simulink model "model2"  (R2022b)
settings: Solver=VariableStepAuto  StartTime=0.0  StopTime=20  RelTol=1e-3
settings Model: Creator=jim  LastModifiedBy=jim

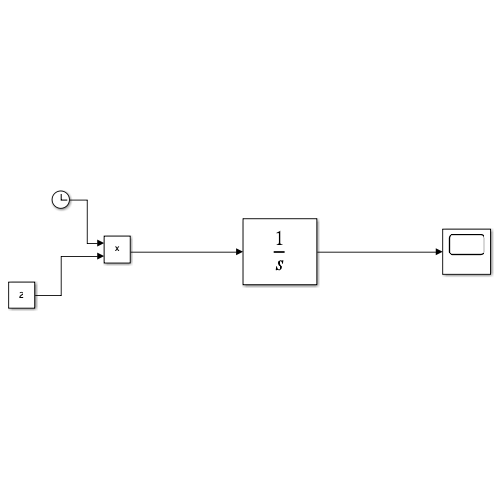
[thumbnail: Simulink's stored preview of the top-level diagram]
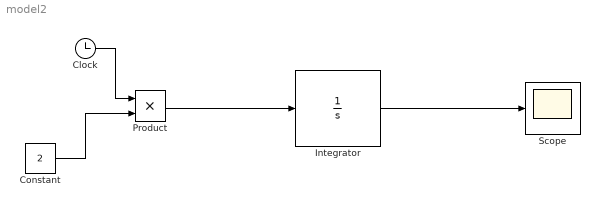
== system model2 ==
  Clock : Clock
  Constant : Constant  Value=2
  Integrator : Integrator
  Product : Product
  Scope : Scope
  wires:
  Clock/1 -> Product/1
  Constant/1 -> Product/2
  Product/1 -> Integrator/1
  Integrator/1 -> Scope/1
